simulink model "Diagrama_distancia"  (R2017b)
settings: Solver=VariableStepAuto  StartTime=0.0  StopTime=100  RelTol=1e-3
values from neighbouring files (symbols this model uses):
  J = 0.0050804    [Controle_de_distancia.m]
  K = 0.087    [Controle_de_distancia.m]    (also in Diagrama_teste.mat)
  La = 0.00015    [Controle_de_distancia.m]    (also in Diagrama_teste.mat)
  m = 1    [Controle_de_distancia.m]    (also in Diagrama_teste.mat)
  R = 0.05    [Controle_de_distancia.m]    (also in Diagrama_teste.mat = 0.2)
  R_l = 3    [Controle_de_distancia.m]    (also in Diagrama_teste.mat)
  R_t = 9    [Controle_de_distancia.m]    (also in Diagrama_teste.mat)
  Ra = 0.1501    [Controle_de_distancia.m]    (also in Diagrama_teste.mat)
  V_ref = 3.3    [Controle_de_distancia.m]    (also in Diagrama_teste.mat)
settings Model: Creator=Victor  LastModifiedBy=Victor

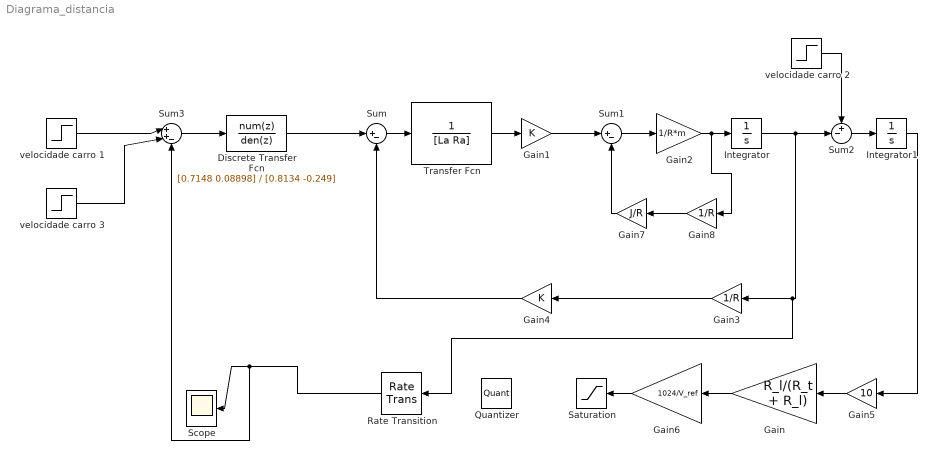
== system Diagrama_distancia ==
  Discrete Transfer Fcn : DiscreteTransferFcn  Numerator=[0.7148 0.08898]  Denominator=[0.8134 -0.249]  SampleTime=1.25
  Gain : Gain  Gain=R_l/(R_t + R_l)
  Gain1 : Gain  Gain=K
  Gain2 : Gain  Gain=1/R*m
  Gain3 : Gain  Gain=1/R
  Gain4 : Gain  Gain=K
  Gain5 : Gain  Gain=10
  Gain6 : Gain  Gain=1024/V_ref
  Gain7 : Gain  Gain=J/R
  Gain8 : Gain  Gain=1/R
  Integrator : Integrator
  Integrator1 : Integrator  InitialCondition=1  LimitOutput=on  LowerSaturationLimit=0
  Quantizer : Quantizer  QuantizationInterval=1.25
  Rate Transition : RateTransition  OutPortSampleTimeMultiple=1.25  OutPortSampleTime=1.25
  Saturation : Saturate  UpperLimit=1024  LowerLimit=0
  Scope : Scope
  Sum : Sum  Inputs=|+-
  Sum1 : Sum  Inputs=|+-
  Sum2 : Sum  Inputs=+-|
  Sum3 : Sum  Inputs=|++-
  Transfer Fcn : TransferFcn  Denominator=[La Ra]
  velocidade carro 1 : Step  Time=0.5  After=0.87  SampleTime=0
  velocidade carro 2 : Step  Time=0.5  After=0  SampleTime=0
  velocidade carro 3 : Step  Time=50  After=0.95  SampleTime=0
  wires:
  Sum/1 -> Transfer Fcn/1
  Gain1/1 -> Sum1/1
  Sum1/1 -> Gain2/1
  Gain3/1 -> Gain4/1
  Gain4/1 -> Sum/2
  Transfer Fcn/1 -> Gain1/1
  Gain2/1 -> Gain8/1, Integrator/1
  Sum2/1 -> Integrator1/1
  velocidade carro 2/1 -> Sum2/1
  Integrator1/1 -> Gain5/1
  Gain5/1 -> Gain/1
  Gain/1 -> Gain6/1
  Gain6/1 -> Saturation/1
  Gain8/1 -> Gain7/1
  Gain7/1 -> Sum1/2
  Integrator/1 -> Sum2/2, Rate Transition/1, Gain3/1
  velocidade carro 1/1 -> Sum3/1
  velocidade carro 3/1 -> Sum3/2
  Rate Transition/1 -> Sum3/3, Scope/1
  Discrete Transfer Fcn/1 -> Sum/1
  Sum3/1 -> Discrete Transfer Fcn/1
